simulink model "DR18E_Testpult"  (R2017a)
settings: Solver=ode1  StartTime=0.0  StopTime=Inf  FixedStep=0.001  RelTol=1e-3
PostLoadFcn:
  | , if any(exist('dsrtsu_mdlpostloadfcn', 'file') == [2, 3, 6]), try dsrtsu_mdlpostloadfcn('Execute', bdroot); catch fprintf('Error in PostLoadFcn (dsrtsu_mdlpostloadfcn) for model "%s":\n %s\n', bdroot, lasterr); end, end,
model workspace: external: MATLAB File C:\Users\DeltaRacing\Documents\dSPACE\MABX_DR18E\Model\DR18E_MABX_Parameter.m (data not in the file)
values from neighbouring files (symbols this model uses):
  am = 1/Ts    (= 1)    [DR18E_MABX_Parameter.m]
  bm = K/Ts    (= 0.05)    [DR18E_MABX_Parameter.m]
  cf = 41350    [DR18E_MABX_Parameter.m]
  cr = 41350    [DR18E_MABX_Parameter.m]
  Derating_HV_Battery_Kapa = 1    [DR18E_MABX_Parameter.m]
  Derating_Start_km = 16    [DR18E_MABX_Parameter.m]
  Drive_Mode = 0    [DR18E_MABX_Parameter.m]
  g = 1    [DR18E_MABX_Parameter.m]
  Gas_Modus = 2    [DR18E_MABX_Parameter.m]
  HV_Power_max = 80    [DR18E_MABX_Parameter.m]
  i_Getriebe = 3.3    [DR18E_MABX_Parameter.m]
  i_Lenkgetriebe = 4.32    [DR18E_MABX_Parameter.m]
  K_SET = 1    [DR18E_MABX_Parameter.m]
  Kapazitaet_HV_Battery_kWh = 6.6    [DR18E_MABX_Parameter.m]
  KW_T_Soll = 37    [DR18E_MABX_Parameter.m]
  lf = 1.2    [DR18E_MABX_Parameter.m]
  lr = 1.15    [DR18E_MABX_Parameter.m]
  m = 310    [DR18E_MABX_Parameter.m]
  M_max = 150    [DR18E_MABX_Parameter.m]
  Power_Limit_onoff = 0    [DR18E_MABX_Parameter.m]
  Reifenradius = 0.2351    [DR18E_MABX_Parameter.m]
  Strecke_Endu_km = 22    [DR18E_MABX_Parameter.m]
  TC_Decr_Gas = 0.00005    (= 5e-05)    [DR18E_MABX_Parameter.m]
  TC_Derivative = 0.4    [DR18E_MABX_Parameter.m]
  TC_Incr_Gas = 0.005    [DR18E_MABX_Parameter.m]
  TC_On = 0    [DR18E_MABX_Parameter.m]
  TC_Relay_Off = 0.065    [DR18E_MABX_Parameter.m]
  TC_Relay_On = 0.07    [DR18E_MABX_Parameter.m]
  TV_Mode = 2    [DR18E_MABX_Parameter.m]
  TV_On = 0    [DR18E_MABX_Parameter.m]
  TV_Override = 1    [DR18E_MABX_Parameter.m]
  y = 0.8    [DR18E_MABX_Parameter.m]
undefined symbols (not defined in the file or in its folder): D, DiscIntNeverNeededParam, I, K_OL, P
libraries: simulink x288, rtican x105, rtiusbflightreclib x40, rti1401lib_dio_type3 x10, simulink_extras x10, rti1401lib_adc_type4 x8, rti1401lib_II_base x7
(part 7 of 28)

== system DR18E_Testpult/Eingabe Fahrzeug/Gyro ==
  note: gyro zero offset changed from -4.2 to 0
  Bit-->deg/s : Gain
  Bus Creator : BusCreator  Inputs=3
  Errorfield : Gain
  FlightRecorder4 : Subsystem
  Gyro Timeout : Constant  Value=1000
  Gyro Zero Offset : Constant  Value=0
  RX Timeout Detection : Subsystem
  Sum : Sum  Inputs=-+|
  Yaw_Rate : rtican/RTICAN Receive (RX)   Reserved1=[]  Reserved2=[]  Reserved3=[]  Reserved4=[]  SfcnMessage=[]  Msg_Struct=[]  BoardTypeNo=[]  BoardNo=[]  ChannelNo=[]  Parameters=[]  DialogFcn=[]  UnitName=[]  Revision=[]  UnitValues=[]  DSProperties=struct('RTI',struct('Version',uint32(5),'BlockType',struct('isSLSource',uint8(1),'isSLSink',uint8(1),'isHWSource',uint8(0),'isHWSink',uint8(0),'isSetup',uint8(0),'isInline',uint8(1),'isNonInline',uint8(0),'isInterrupt',uint8(0),'isChannelwise',uint8(0)),'IOBoardType','RTICAN','UnitType','MESSAGE','Identifier','RX','DialogType','MSVC','BlockSet','RTICAN','SlaveProcessor','CAN'))  RTIBlockInterface=struct('OutputPortsWidth',int32([1 1 1 1 1]),'OutputPortsActive',[1 1 1 1 1],'OutputPortsName',{{'Yaw_Z','Yaw_Z_Error',['RX status'],['RX time'],['RX delta time']}},'OutputPortsDataType',{{'SS_DOUBLE','SS_DOUBLE','SS_DOUBLE','SS_DOUBLE','SS_DOUBLE'}},'OutputPortsLabel',{{'Yaw_Z','Yaw_Z_Error','','',''}},'OutputPortsLabelMode','ON','InputPortsWidth',int32(0),'InputPortsActive',0,'DialogFcn','rtican_message_interface_gui','BlockDisplay',{{'','center'}},'IconTransparency','on','ParameterTunableNames',{{}},'InitLevel',3,'BlockName',struct('Token',{{'Yaw_Rate'}}),'SampleTime',{{-1}},'TriggerPort',{{'none'}},'EnablePort',{{'none'}})  RTIBlockParameters=struct('BoardTypeNo',{{1,'OFF',[]}},'BoardNo',{{2,'ON',[1 16]}},'ChannelNo',{{1,'ON',[1 2]}},'Parameters',{{struct('DataFileSupport',struct('DataFileSelectedMaster',1,'DataFileSelectedLocal',1,'DataFileName','c:\users\deltaracing\documents\canoe\dr18e\dbc\dr18e.dbc|','DataFileDate',['16-Feb-2019 13:23:09'],'SelectedFile','..\..\..\canoe\dr18e_test\dr18e\dbc\dr18e.dbc','InterfaceFcn','rtican_dbc_file_parser'),'Options',struct('StatusSelected',1,'TimeSelected',1,'DeltaTimeSelected',1,'BytePortSelected',0,'MessageLengthSelected',0,'TriggerPort',struct('Selected',0,'TriggerType',0),'UserCoding',struct('Selected',0,'InterfaceFile','UserDecodingFile','FcnName','UserDecodeFcn','InportSelected',0,'InportWidth',1,'OutportSelected',0,'OutportWidth',1),'EnablePortSelected',0,'SignalOnPortnameSelected',1,'UseRXService',0),'Message',struct('MsgOnBlocknameSelected',1,'MsgName','Yaw_Rate','MsgIdFormat',0,'MsgId',307,'MsgLength',3,'NumSignals',2,'SampleTime',-1,'Signal',struct('SgnName',{'Yaw_Z','Yaw_Z_Error'},'SgnStartBit',{0,16},'SgnLength',{16,8},'ByteLayout',{0,0},'Factor',{0.00875,1},'Offset',{0,0},'SgnComment',{['Umrechnung Offset beachten'],''},'SgnUnit',{'°/s',''},'Min',{0,0},'Max',{0,0},'SgnType',{0,0},'SLDataType',{'SS_DOUBLE','SS_DOUBLE'},'DataType',{1,1},'ModeValue',{-1,-1}),'MsgIdNumFormat',0,'MsgComment',{{''}}),'Version',1.2,'general',struct('isFromLib',0)),'OFF',[]}},'GroupId',{{struct('Group',{{'RTICAN'}},'No',1,'Behavior',{{'NAMECHANGE'}},'BlockType',{{'SINK'}},'NameChangeFlag',0),'OFF',[]}},'SFcnRTICANMessage',{{struct('MsgType','RX','SFcnPortType','Scalar','MsgName','Yaw_Rate','MsgIdFormat','STD','MsgId',307,'MsgLength',3,'NumSignals',2,'SampleTime',-1,'Signal',struct('SgnName',{'Yaw_Z','Yaw_Z_Error'},'SgnStartBit',{0,16},'SgnLength',{16,8},'ByteLayout',{['little endian'],['little endian']},'Factor',{0.00875,1},'Offset',{0,0},'SgnType',{'standard','standard'},'SLDataType',{'SS_DOUBLE','SS_DOUBLE'},'DataType',{['signed int'],['signed int']},'ModeValue',{-1,-1}),'StatusSelected','yes','TimeSelected','yes','DeltaTimeSelected','yes','BytePortSelected','no','MessageLengthSelected','no','TriggerPort',struct('Selected','no','TriggerType',0),'UserCoding',struct('Selected','no','InterfaceFile','UserDecodingFile','FcnName','UserDecodeFcn','InportSelected','no','InportWidth',1,'OutportSelected','no','OutportWidth',1),'EnablePortSelected','no','UseRXService','no','BoardType','DS1','BoardNo',2,'ControllerNo',1),'OFF',[]}},'TLCFileName',{{'rtican_rx_message','OFF',[]}})  RTISFcnParameters=struct('SFcnRTICANMessage','struct','TLCFileName','char')  RTIBlockParaDefault=struct('BoardTypeNo',4302,'BoardNo',1,'ChannelNo',1,'Parameters',struct('DataFileSupport',struct('DataFileSelectedMaster',0,'DataFileSelectedLocal',0,'DataFileName','','DataFileDate','','SelectedFile',['<no file selected>']),'Options',struct('StatusSelected',1,'TimeSelected',1,'DeltaTimeSelected',1,'BytePortSelected',0,'MessageLengthSelected',0,'TriggerPort',struct('Selected',0,'TriggerType','rising'),'UserCoding',struct('Selected',0,'InterfaceFile','UserDecodingFile','FcnName','UserDecodeFcn','InportSelected',0,'InportWidth',1,'OutportSelected',0,'OutportWidth',1),'EnablePortSelected',0,'SignalOnPortnameSelected',1,'UseRXService',0),'Message',struct('MsgOnBlocknameSelected',0,'MsgName',['RX Message'],'MsgIdFormat',0,'MsgId',100,'MsgLength',8,'NumSignals',1,'SampleTime',-1,'Signal',struct('SgnName',['RX signal'],'SgnStartBit',0,'SgnLength',8,'SgnType',0,'ModeValue',-1,'DataType',0,'SLDataType','SS_DOUBLE','ByteLayout',0,'Factor',1,'Offset',0,'Min',0,'Max',255,'SgnComment',{{}},'SgnUnit',''),'MsgIdNumFormat',0,'MsgComment',{{''}}),'Version',1.2,'general',struct('isFromLib',1)),'GroupId',struct('Group',{{'RTICAN'}},'No',1,'Behavior',{{'NAMECHANGE'}},'BlockType',{{'SINK'}},'NameChangeFlag',0),'SFcnRTICANMessage',struct('MsgType','RX','MsgName',['RX Message'],'MsgIdFormat','STD','MsgId',100,'MsgLength',8,'NumSignals',1,'SampleTime',-1,'Signal',struct('SgnName',['RX signal'],'SgnStartBit',0,'SgnLength',8,'SgnType','standard','ModeValue',-1,'DataType',['unsigned int'],'ByteLayout',['little endian'],'SLDataType','SS_DOUBLE','Factor',1,'Offset',0),'StatusSelected','yes','TimeSelected','yes','DeltaTimeSelected','yes','BytePortSelected','no','MessageLengthSelected','no','EnablePortSelected','no','UserCoding',struct('Selected','no','InterfaceFile','UserDecodingFile','FcnName','UserDecodeFcn','InportSelected','no','InportWidth',1,'OutportSelected','no','OutportWidth',1),'TriggerPort',struct('Selected','no','TriggerType','rising'),'UseRXService','no','BoardType','DS4302','BoardNo',1,'ControllerNo',1,'SFcnPortType','Scalar'),'TLCFileName','rtican_rx_message')
      settings: AttributesFormatString=Group Id: RTICAN1\n  SourceProductName=dSPACE RTI CAN Blockset
  Gyro : Outport
  wires:
  Yaw_Rate/3 -> RX Timeout Detection/1(RX status)
  Bit-->deg/s/1 -> Sum/2
  Errorfield/1 -> Bus Creator/2  "Yaw_Z_Error"
  Bus Creator/1 -> Gyro/1  "RX_Gyro_deg/s"
  Gyro Timeout/1 -> RX Timeout Detection/2(Timeout (n Samples))
  RX Timeout Detection/1(RX Timeout Error) -> Bus Creator/3  "RX Timeout Error"
  Sum/1 -> Bus Creator/1, FlightRecorder4/1(In1)  "Yaw_Z"
  Gyro Zero Offset/1 -> Sum/1
  Yaw_Rate/1 -> Bit-->deg/s/1  "Yaw_Z"
  Yaw_Rate/2 -> Errorfield/1  "Yaw_Z_Error"

== system DR18E_Testpult/Eingabe Fahrzeug/Inverter Feedback Messages ==
  Bus Creator : BusCreator  Inputs=2
  Bus Creator1 : BusCreator  Inputs=10
  Bus Creator2 : BusCreator  Inputs=10
  "Istwerte Umrichter 1 empfangen " : Subsystem
  Istwerte Umrichter 2 empfangen : Subsystem
  Out1 : Outport
  wires:
  Istwerte Umrichter 2 empfangen/1(Motor_Temp) -> Bus Creator1/1  "Mot_Temp"
  Istwerte Umrichter 2 empfangen/2(Drehzahl 1_min) -> Bus Creator1/2  "Drehzahl_1min"
  Istwerte Umrichter 2 empfangen/3(Iq_A) -> Bus Creator1/3  "Iq_A"
  Bus Creator1/1 -> Bus Creator/2  "U2"
  Istwerte Umrichter 2 empfangen/4(P_W) -> Bus Creator1/4  "P_W"
  Istwerte Umrichter 2 empfangen/5(Mmot_Nm) -> Bus Creator1/5  "Mmot_Nm"
  Istwerte Umrichter 2 empfangen/6(IRMS_A) -> Bus Creator1/6  "IRMS_A"
  Istwerte Umrichter 2 empfangen/7(UDC) -> Bus Creator1/7  "UDC_V"
  Istwerte Umrichter 2 empfangen/8(Sammelwarnung) -> Bus Creator1/8  "Sammelwarnung"
  Istwerte Umrichter 2 empfangen/9(Sammelstörung) -> Bus Creator1/9  "Sammelstörung"
  "Istwerte Umrichter 1 empfangen "/1(Motor_Temp) -> Bus Creator2/1  "Mot_Temp"
  "Istwerte Umrichter 1 empfangen "/2(Drehzahl 1_min) -> Bus Creator2/2  "Drehzahl_1min"
  "Istwerte Umrichter 1 empfangen "/3(Iq_A) -> Bus Creator2/3  "Iq_A"
  "Istwerte Umrichter 1 empfangen "/4(P_W) -> Bus Creator2/4  "P_W"
  "Istwerte Umrichter 1 empfangen "/5(Mmot_Nm) -> Bus Creator2/5  "Mmot_Nm"
  "Istwerte Umrichter 1 empfangen "/6(IRMS_A) -> Bus Creator2/6  "IRMS_A"
  "Istwerte Umrichter 1 empfangen "/7(UDC) -> Bus Creator2/7  "UDC_V"
  "Istwerte Umrichter 1 empfangen "/8(Sammelwarnung) -> Bus Creator2/8  "Sammelwarnung"
  "Istwerte Umrichter 1 empfangen "/9(Sammelstörung) -> Bus Creator2/9  "Sammelstörung"
  Bus Creator2/1 -> Bus Creator/1  "U1"
  Istwerte Umrichter 2 empfangen/10(InverterTemp) -> Bus Creator1/10  "InverterTemp"
  "Istwerte Umrichter 1 empfangen "/10(InverterTemp) -> Bus Creator2/10  "InverterTemp"
  Bus Creator/1 -> Out1/1  "Umrichter"

== system DR18E_Testpult/Eingabe Fahrzeug/Lenkwinkelgeber ==
  Bus Creator : BusCreator  Inputs=4
  FlightRecorder : Subsystem
  Gyro Timeout : Constant  Value=1000
  RX Timeout Detection : Subsystem
  Steering : rtican/RTICAN Receive (RX)   Reserved1=[]  Reserved2=[]  Reserved3=[]  Reserved4=[]  SfcnMessage=[]  Msg_Struct=[]  BoardTypeNo=[]  BoardNo=[]  ChannelNo=[]  Parameters=[]  DialogFcn=[]  UnitName=[]  Revision=[]  UnitValues=[]  DSProperties=struct('RTI',struct('Version',uint32(5),'BlockType',struct('isSLSource',uint8(1),'isSLSink',uint8(1),'isHWSource',uint8(0),'isHWSink',uint8(0),'isSetup',uint8(0),'isInline',uint8(1),'isNonInline',uint8(0),'isInterrupt',uint8(0),'isChannelwise',uint8(0)),'IOBoardType','RTICAN','UnitType','MESSAGE','Identifier','RX','DialogType','MSVC','BlockSet','RTICAN','SlaveProcessor','CAN'))  RTIBlockInterface=struct('OutputPortsWidth',int32([1 1 1 1]),'OutputPortsActive',[1 1 1 1],'OutputPortsName',{{'Steering',['RX status'],['RX time'],['RX delta time']}},'OutputPortsDataType',{{'SS_DOUBLE','SS_DOUBLE','SS_DOUBLE','SS_DOUBLE'}},'OutputPortsLabel',{{'Steering','','',''}},'OutputPortsLabelMode','ON','InputPortsWidth',int32(0),'InputPortsActive',0,'DialogFcn','rtican_message_interface_gui','BlockDisplay',{{'','center'}},'IconTransparency','on','ParameterTunableNames',{{}},'InitLevel',3,'BlockName',struct('Token',{{'Steering'}}),'SampleTime',{{-1}},'TriggerPort',{{'none'}},'EnablePort',{{'none'}})  RTIBlockParameters=struct('BoardTypeNo',{{1,'OFF',[]}},'BoardNo',{{2,'ON',[1 16]}},'ChannelNo',{{1,'ON',[1 2]}},'Parameters',{{struct('DataFileSupport',struct('DataFileSelectedMaster',1,'DataFileSelectedLocal',1,'DataFileName','c:\users\deltaracing\documents\canoe\dr18e\dbc\dr18e.dbc|','DataFileDate',['16-Feb-2019 13:23:09'],'SelectedFile','..\..\..\canoe\dr18e_test\dr18e\dbc\dr18e.dbc','InterfaceFcn','rtican_dbc_file_parser'),'Options',struct('StatusSelected',1,'TimeSelected',1,'DeltaTimeSelected',1,'BytePortSelected',0,'MessageLengthSelected',0,'TriggerPort',struct('Selected',0,'TriggerType',0),'UserCoding',struct('Selected',0,'InterfaceFile','UserDecodingFile','FcnName','UserDecodeFcn','InportSelected',0,'InportWidth',1,'OutportSelected',0,'OutportWidth',1),'EnablePortSelected',0,'SignalOnPortnameSelected',1,'UseRXService',0),'Message',struct('MsgOnBlocknameSelected',1,'MsgName','Steering','MsgIdFormat',0,'MsgId',416,'MsgLength',2,'NumSignals',1,'SampleTime',-1,'Signal',struct('SgnName','Steering','SgnStartBit',0,'SgnLength',16,'ByteLayout',0,'Factor',0.1,'Offset',0,'SgnComment','','SgnUnit','°','Min',0,'Max',0,'SgnType',0,'SLDataType','SS_DOUBLE','DataType',1,'ModeValue',-1),'MsgIdNumFormat',0,'MsgComment',{{''}}),'Version',1.2,'general',struct('isFromLib',0)),'OFF',[]}},'GroupId',{{struct('Group',{{'RTICAN'}},'No',1,'Behavior',{{'NAMECHANGE'}},'BlockType',{{'SINK'}},'NameChangeFlag',0),'OFF',[]}},'SFcnRTICANMessage',{{struct('MsgType','RX','SFcnPortType','Scalar','MsgName','Steering','MsgIdFormat','STD','MsgId',416,'MsgLength',2,'NumSignals',1,'SampleTime',-1,'Signal',struct('SgnName','Steering','SgnStartBit',0,'SgnLength',16,'ByteLayout',['little endian'],'Factor',0.1,'Offset',0,'SgnType','standard','SLDataType','SS_DOUBLE','DataType',['signed int'],'ModeValue',-1),'StatusSelected','yes','TimeSelected','yes','DeltaTimeSelected','yes','BytePortSelected','no','MessageLengthSelected','no','TriggerPort',struct('Selected','no','TriggerType',0),'UserCoding',struct('Selected','no','InterfaceFile','UserDecodingFile','FcnName','UserDecodeFcn','InportSelected','no','InportWidth',1,'OutportSelected','no','OutportWidth',1),'EnablePortSelected','no','UseRXService','no','BoardType','DS1','BoardNo',2,'ControllerNo',1),'OFF',[]}},'TLCFileName',{{'rtican_rx_message','OFF',[]}})  RTISFcnParameters=struct('SFcnRTICANMessage','struct','TLCFileName','char')  RTIBlockParaDefault=struct('BoardTypeNo',4302,'BoardNo',1,'ChannelNo',1,'Parameters',struct('DataFileSupport',struct('DataFileSelectedMaster',0,'DataFileSelectedLocal',0,'DataFileName','','DataFileDate','','SelectedFile',['<no file selected>']),'Options',struct('StatusSelected',1,'TimeSelected',1,'DeltaTimeSelected',1,'BytePortSelected',0,'MessageLengthSelected',0,'TriggerPort',struct('Selected',0,'TriggerType','rising'),'UserCoding',struct('Selected',0,'InterfaceFile','UserDecodingFile','FcnName','UserDecodeFcn','InportSelected',0,'InportWidth',1,'OutportSelected',0,'OutportWidth',1),'EnablePortSelected',0,'SignalOnPortnameSelected',1,'UseRXService',0),'Message',struct('MsgOnBlocknameSelected',0,'MsgName',['RX Message'],'MsgIdFormat',0,'MsgId',100,'MsgLength',8,'NumSignals',1,'SampleTime',-1,'Signal',struct('SgnName',['RX signal'],'SgnStartBit',0,'SgnLength',8,'SgnType',0,'ModeValue',-1,'DataType',0,'SLDataType','SS_DOUBLE','ByteLayout',0,'Factor',1,'Offset',0,'Min',0,'Max',255,'SgnComment',{{}},'SgnUnit',''),'MsgIdNumFormat',0,'MsgComment',{{''}}),'Version',1.2,'general',struct('isFromLib',1)),'GroupId',struct('Group',{{'RTICAN'}},'No',1,'Behavior',{{'NAMECHANGE'}},'BlockType',{{'SINK'}},'NameChangeFlag',0),'SFcnRTICANMessage',struct('MsgType','RX','MsgName',['RX Message'],'MsgIdFormat','STD','MsgId',100,'MsgLength',8,'NumSignals',1,'SampleTime',-1,'Signal',struct('SgnName',['RX signal'],'SgnStartBit',0,'SgnLength',8,'SgnType','standard','ModeValue',-1,'DataType',['unsigned int'],'ByteLayout',['little endian'],'SLDataType','SS_DOUBLE','Factor',1,'Offset',0),'StatusSelected','yes','TimeSelected','yes','DeltaTimeSelected','yes','BytePortSelected','no','MessageLengthSelected','no','EnablePortSelected','no','UserCoding',struct('Selected','no','InterfaceFile','UserDecodingFile','FcnName','UserDecodeFcn','InportSelected','no','InportWidth',1,'OutportSelected','no','OutportWidth',1),'TriggerPort',struct('Selected','no','TriggerType','rising'),'UseRXService','no','BoardType','DS4302','BoardNo',1,'ControllerNo',1,'SFcnPortType','Scalar'),'TLCFileName','rtican_rx_message')
      settings: AttributesFormatString=Group Id: RTICAN1\n  SourceProductName=dSPACE RTI CAN Blockset
  LenkwinkelgeberOut : Outport
  wires:
  Bus Creator/1 -> LenkwinkelgeberOut/1  "RX_Lenkwinkel"
  Steering/2 -> RX Timeout Detection/1(RX status)
  Gyro Timeout/1 -> RX Timeout Detection/2(Timeout (n Samples))
  RX Timeout Detection/1(RX Timeout Error) -> Bus Creator/2  "RX Timeout Error"
  Steering/1 -> Bus Creator/1, FlightRecorder/1(In1)  "Steering"

== system DR18E_Testpult/Eingabe Fahrzeug/MicroAutoBox ==
  AI : Subsystem
  Beschleunigungssensor : Subsystem
  Bus Creator : BusCreator  Inputs=3
  DI : Subsystem
  MicroAutoBox : Outport
  wires:
  Bus Creator/1 -> MicroAutoBox/1  "MicroAutoBox"
  DI/1(DI) -> Bus Creator/1
  AI/1(AI) -> Bus Creator/2
  Beschleunigungssensor/1(Beschleunigungssensor) -> Bus Creator/3
